simulink model "traj_track_output_error_feedback_ctrl"  (R2025b)
settings: Solver=VariableStepAuto  StartTime=0.0  StopTime=35  RelTol=1e-3
libraries: simulink x1, robotmobilelib x1
settings Model: Creator=alessandrochinello  LastModifiedBy=mattc

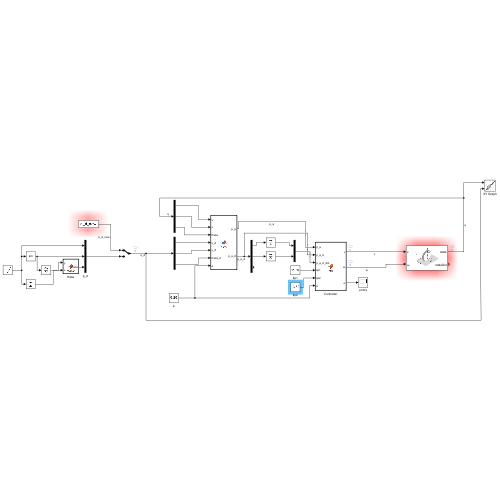
[thumbnail: Simulink's stored preview of the top-level diagram]
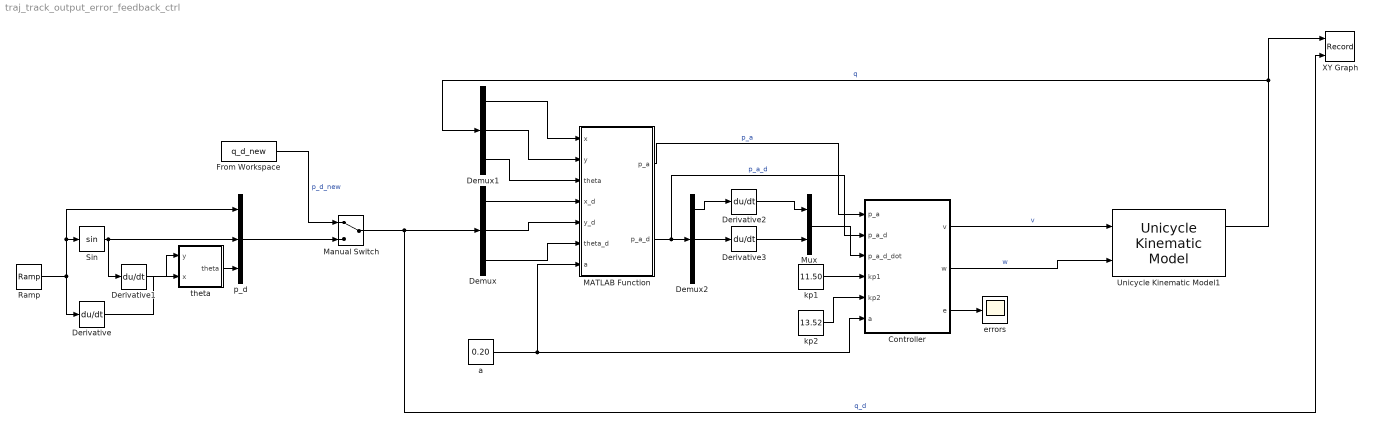
== system traj_track_output_error_feedback_ctrl ==
  Controller : MATLAB Function  TreatAsAtomicUnit=on
  Demux : Demux  Outputs=3
  Demux1 : Demux  Outputs=3
  Demux2 : Demux  Outputs=3
  Derivative{,1..3} (4 alike) : Derivative
  From Workspace : FromWorkspace  VariableName=q_d_new
  MATLAB Function : MATLAB Function  TreatAsAtomicUnit=on
  Manual Switch : ManualSwitch
  Mux : Mux  Inputs=2
  Ramp : simulink/Sources/Ramp  slope=1  start=0  InitialOutput=0
  Sin : Trigonometry
  Unicycle Kinematic Model1 : robotmobilelib/Unicycle Kinematic Model  VehicleInputs=Vehicle Speed & Heading Angular Velocity  WheelRadius=0.1  WheelSpeedRange=[-Inf Inf]  InitialState=q0  SimulateUsing=Interpreted execution
  XY Graph : Record  NumPorts=2.0  FileSettingsInternal="{\"entries\":[{\"content\":{\"excelSettings\":{\"content\":{},\"type\":\"Streamout.ExcelSettings\"},\"parquetSettings\":{\"content\":{},\"type\":\"Streamout.ParquetSettings\"}},\"type\":\"Streamout.FileSettingStorage\",\"uuid\":\"\"}],\"packageUris\":[\"http:\\/\\/schema.mathworks.com\\/mf0\\/streamout_blocks\\/R2020a\"],\"version\":\"1.0\"}"  FrameSettings=[0, 0]  Layout=[1 1]  SignalsInternal="{\"entries\":[{\"content\":{\"signals\":[{\"content\":{\"blockPath\":[],\"dimensions\":[3],\"domain\":\"\",\"hasChildren\":true,\"lineColor\":\"#ff13a6\",\"lineWidth\":2,\"port\":1,\"sid\":[\"\"],\"signalID\":1,\"signalName\":\"q\"},\"type\":\"RecordBlkView.Signal\",\"uuid\":\"\"},{\"content\":{\"blockPath\":[],\"channel\":[1],\"dimensions\":[3],\"domain\":\"\",\"lineColor\":\"#22b573\",\"lineWidth\":2,\"parentID\":1,\"plots\":[ 1 ],\"port\":1,\"sid\":[\"\"],\"signalID\":2,\"signalName\":\"q\"},\"type\":\"RecordBlkView.Signal\",\"uuid\":\"\"},{\"content\":{\"blockPath\":[],\"dimensions\":[3],\"domain\":\"\",\"hasChildren\":true,\"lineColor\":\"#22b573\",\"lineWidth\":2,\"port\":2,\"sid\":[\"\"],\"signalID\":3,\"signalName\":\"q_d\"},\"type\":\"RecordBlkView.Signal\",\"uuid\":\"\"},{\"content\":{\"blockPath\":[],\"channel\":[1],\"dimensions\":[3],\"domain\":\"\",\"lineColor\":\"#d95319\",\"lineWidth\":2,\"parentID\":3,\"plots\":[ 1 ],\"port\":2,\"sid\":[\"\"],\"signalID\":4,\"signalName\":\"q_d\"},\"type\":\"RecordBlkView.Signal\",\"uuid\":\"\"},{\"content\":{\"blockPath\":[],\"channel\":[2],\"dimensions\":[3],\"domain\":\"\",\"lineColor\":\"#a2142f\",\"lineWidth\":2,\"parentID\":1,\"plots\":[ 1 ],\"port\":1,\"sid\":[\"\"],\"signalID\":5,\"signalName\":\"q\"},\"type\":\"RecordBlkView.Signal\",\"uuid\":\"\"},{\"content\":{\"blockPath\":[],\"channel\":[3],\"dimensions\":[3],\"domain\":\"\",\"lineColor\":\"#139fff\",\"lineWidth\":2,\"parentID\":1,\"port\":1,\"sid\":[\"\"],\"signalID\":6,\"signalName\":\"q\"},\"type\":\"RecordBlkView.Signal\",\"uuid\":\"\"},{\"content\":{\"blockPath\":[],\"channel\":[2],\"dimensions\":[3],\"domain\":\"\",\"lineColor\":\"#ff6929\",\"lineWidth\":2,\"parentID\":3,\"plots\":[ 1 ],\"port\":2,\"sid\":[\"\"],\"signalID\":7,\"signalName\":\"q_d\"},\"type\":\"RecordBlkView.Signal\",\"uuid\":\"\"},{\"content\":{\"blockPath\":[],\"channel\":[3],\"dimensions\":[3],\"domain\":\"\",\"lineColor\":\"#b746ff\",\"lineWidth\":2,\"parentID\":3,\"port\":2,\"sid\":[\"\"],\"signalID\":8,\"signalName\":\"q_d\"},\"type\":\"RecordBlkView.Signal\",\"uuid\":\"\"}]},\"type\":\"RecordBlkView.InputSignals\",\"uuid\":\"\"}],\"packageUris\":[\"http:\\/\\/schema.mathworks.com\\/mf0\\/streamout_blocks\\/R2020a\"],\"version\":\"1.0\"}"  VisualizationBindings="{\"xyplotplugin\":{\"info\":[{\"series\":[{\"bindingParametersList\":[{\"parameter\":\"X-Axis\",\"signalID\":4,\"signalName\":\"q_d(1)\"},{\"parameter\":\"Y-Axis\",\"signalID\":7,\"signalName\":\"q_d(2)\"}],\"seriesID\":0},{\"bindingParametersList\":[{\"parameter\":\"X-Axis\",\"signalID\":2,\"signalName\":\"q(1)\"},{\"parameter\":\"Y-Axis\",\"signalID\":5,\"signalName\":\"q(2)\"}],\"seriesID\":1}],\"subplotID\":1}]}}"  CompatibilityTag=XY
  a : Constant  Value=0.20
  errors : Scope
      settings: ActiveDisplayYMinimum=-0.80222452395317112  ActiveDisplayYMaximum=0.0900014086361547
  kp1 : Constant  Value=11.50
  kp2 : Constant  Value=13.52
  p_d : Mux  Inputs=3
  theta : MATLAB Function  TreatAsAtomicUnit=on
  wires:
  Controller/2(w) -> Unicycle Kinematic Model1/2  "w"
  Demux2/2 -> Derivative3/1
  From Workspace/1 -> Manual Switch/1  "p_d_new"
  kp2/1 -> Controller/5(kp2)
  Derivative3/1 -> Mux/2
  Mux/1 -> Controller/3(p_a_d_dot)
  Ramp/1 -> Sin/1, p_d/1, Derivative/1
  Derivative2/1 -> Mux/1
  MATLAB Function/2(p_a_d) -> Demux2/1, Controller/2(p_a_d)  "p_a_d"
  kp1/1 -> Controller/4(kp1)
  Demux/3 -> MATLAB Function/6(theta_d)
  Demux/2 -> MATLAB Function/5(y_d)
  a/1 -> MATLAB Function/7(a), Controller/6(a)
  Demux/1 -> MATLAB Function/4(x_d)
  Controller/3(e) -> errors/1
  Demux1/2 -> MATLAB Function/2(y)
  Manual Switch/1 -> XY Graph/2, Demux/1  "q_d"
  Unicycle Kinematic Model1/1 -> Demux1/1, XY Graph/1  "q"
  MATLAB Function/1(p_a) -> Controller/1(p_a)  "p_a"
  Demux1/3 -> MATLAB Function/3(theta)
  Demux2/1 -> Derivative2/1
  theta/1(theta) -> p_d/3
  p_d/1 -> Manual Switch/2
  Controller/1(v) -> Unicycle Kinematic Model1/1  "v"
  Demux1/1 -> MATLAB Function/1(x)
  Derivative/1 -> theta/2(x)
  Sin/1 -> Derivative1/1, p_d/2
  Derivative1/1 -> theta/1(y)

== matlab function traj_track_output_error_feedback_ctrl/Controller ==
  data: p_a input; p_a_d input; v output; p_a_d_dot input; w output; e output size=[1,2]; kp1 input; kp2 input; a input
function [v, w, e]= ctrl(p_a , p_a_d, p_a_d_dot, kp1, kp2, a)

% Get desired state
x_a_d = p_a_d(1);
y_a_d = p_a_d(2);

% Get desired velocity state
x_a_d_dot = p_a_d_dot(1);
y_a_d_dot = p_a_d_dot(2);

% If p_a_d_dot is Inf or NaN at the start we put to 0
if ~isfinite(x_a_d_dot), x_a_d_dot = 0; end
if ~isfinite(y_a_d_dot), y_a_d_dot = 0; end

% Get (real) theta
x_a = p_a(1);
y_a = p_a(2);
theta = p_a(3);

% Compute errors (Calcolati tra punto desiderato e punto reale A)
e1 = x_a_d - x_a;
e2 = y_a_d - y_a;

% Control law
v = cos(theta)*(x_a_d_dot + kp1*e1) + sin(theta)*(y_a_d_dot + kp2*e2);
w = -(sin(theta)/a) *(x_a_d_dot + kp1*e1) + (cos(theta)/a)*(y_a_d_dot + kp2*e2);

% Avoid to pass non finite values to kinematics model to the unycicle
if ~isfinite(v), v = 0; end
if ~isfinite(w), w = 0; end

e = [e1 e2];

== matlab function traj_track_output_error_feedback_ctrl/theta ==
  data: y input; x input; theta output
function theta = atan2(y, x)

theta = atan2(y, x);

== matlab function traj_track_output_error_feedback_ctrl/MATLAB Function ==
  data: p_a output; x input; y input; theta input; x_d input; y_d input; theta_d input; p_a_d output size=[1,3]; a input
function [p_a, p_a_d] = p2A(x, y, theta, x_d, y_d, theta_d, a)

% Computing reference trajectory with the com translated
x_a_d = x_d + a * cos(theta_d);
y_a_d = y_d + a * sin(theta_d); 
    

% Computing actual state with the com translated
x_a = x + a * cos(theta);
y_a = y + a * sin(theta);

% Output the P2A transformation
p_a = [x_a, y_a, theta];
p_a_d = [x_a_d, y_a_d, theta_d];
